simulink model "FOC_Motor_Control"  (R2020b)
settings: Solver=FixedStepDiscrete  StartTime=0.0  StopTime=10.0  FixedStep=Fixed_Step_Size  RelTol=1e-3
values from neighbouring files (symbols this model uses):
  Angle = 1.0    [Hall_Flux_FOC_Data.sldd]    (also in Motor_Control_Data.sldd)
  Cosine_table = 1.0 0.99999529 0.99999058 0.99998587 0.99998116 0.99996704 0.99995291 0.99993885 0.99992472 0.99990118 0.99987763 0.99985409 0.9998306 0.99979764 0.99976468 0.99973178 0.99969882 0.99965644 0.99961412 0.99957174 0.99952942 0.99947762 0.99942589 0.99937415 0.99932235 0.9992612 0.99920005 0.99913889 0.99907768 0.99900717 0.99893659 0.99886602 0.99879545 0.99871546 0.99863547 0.99855554 0.99847555 0.    [Hall_Flux_FOC_Data.sldd]    (also in Motor_Control_Data.sldd)
  Flux = 0.0109    [G474_FOC_LADRC.sldd]    (also in G474_FOC_NONOBSERVER.sldd = 0.0109
  HaLL_AngleShift = -0.25    [Hall_Flux_FOC_Data.sldd]
  HaLL_Sector1 = 5.236    [Hall_Flux_FOC_Data.sldd]
  HaLL_Sector2 = 1.0472    [Hall_Flux_FOC_Data.sldd]
  HaLL_Sector3 = 0.0    [Hall_Flux_FOC_Data.sldd]
  HaLL_Sector4 = 3.1415    [Hall_Flux_FOC_Data.sldd]
  HaLL_Sector5 = 4.1888    [Hall_Flux_FOC_Data.sldd]
  HaLL_Sector6 = 2.0944    [Hall_Flux_FOC_Data.sldd]
  HaLL_Timer_T = 1.0E-5    [Hall_Flux_FOC_Data.sldd]
  ID_Ki = 1.3    [Hall_Flux_FOC_Data.sldd]    (also in Motor_Control_Data.sldd = 48.0
  ID_Kp = 0.4    [Hall_Flux_FOC_Data.sldd]    (also in Motor_Control_Data.sldd = 0.84
  inverter = struct    [PMSM_Parameters.m]
  IQ_Ki = 1.6    [Hall_Flux_FOC_Data.sldd]    (also in Motor_Control_Data.sldd = 48.0
  IQ_Kp = 0.4    [Hall_Flux_FOC_Data.sldd]    (also in Motor_Control_Data.sldd = 1.869
  LADRC_b0 = 10000.0    [G474_FOC_LADRC.sldd]    (also in Hall_Flux_FOC_Data.sldd = 80000.0
  LADRC_Omega_c = 100.0    [G474_FOC_LADRC.sldd]    (also in Hall_Flux_FOC_Data.sldd = 80.0
  Ld = 0.0004    [Hall_Flux_FOC_Data.sldd]    (also in Motor_Control_Data.sldd = 0.00014
  Lq = 0.00045    [Hall_Flux_FOC_Data.sldd]    (also in Motor_Control_Data.sldd = 0.0003115
  OPL_Speed = 800.0    [Hall_Flux_FOC_Data.sldd]
  OPL_Time = 2.0    [Hall_Flux_FOC_Data.sldd]
  OPL_Torque = 3.0    [Hall_Flux_FOC_Data.sldd]
  Over_modulation = 0.0    [Hall_Flux_FOC_Data.sldd]    (also in Motor_Control_Data.sldd)
  pll_omega = 5000.0    [G474_FOC_LADRC.sldd]    (also in G474_FOC_NONOBSERVER.sldd)
  pll_xi = 10.0    [G474_FOC_LADRC.sldd]    (also in G474_FOC_NONOBSERVER.sldd)
  Pole_Pairs = 2.0    [Hall_Flux_FOC_Data.sldd]    (also in Motor_Control_Data.sldd = 4.0
  PWM_Frequency = 10000.0    [Hall_Flux_FOC_Data.sldd]    (also in Motor_Control_Data.sldd = 20000.0
  R = 0.405    [Hall_Flux_FOC_Data.sldd]    (also in Motor_Control_Data.sldd = 0.016
  Sine_table = 0.0 0.0015339879 0.0030679768 0.0046019657 0.0061359555 0.0076698866 0.0092038177 0.010737749 0.012271681 0.013805497 0.015339312 0.016873131 0.018406944 0.019940587 0.021474229 0.023007872 0.024541514 0.026074925 0.027608337 0.029141748 0.03067516 0.032208283 0.033741407 0.035274528 0.036807653 0.038340431 0.039873205 0.04140598 0.042938754 0.04447113 0.046003502 0.047535874 0.049068246 0.0506001    [Hall_Flux_FOC_Data.sldd]    (also in Motor_Control_Data.sldd)
  Speed_Ki = 0.06    [Hall_Flux_FOC_Data.sldd]    (also in Motor_Control_Data.sldd = 10.809
  Speed_Kp = 0.002    [Hall_Flux_FOC_Data.sldd]    (also in Motor_Control_Data.sldd = 0.08
  Speed_PI_OutputMax = 3.0    [Hall_Flux_FOC_Data.sldd]    (also in Motor_Control_Data.sldd = 700.0
  Speed_PI_OutputMin = -5.0    [Hall_Flux_FOC_Data.sldd]    (also in Motor_Control_Data.sldd = -700.0
  SpeedFilter_Fn = 0.3    [Hall_Flux_FOC_Data.sldd]    (also in Motor_Control_Data.sldd = 0.2
  TorqueMode = 0.0    [Hall_Flux_FOC_Data.sldd]    (also in Motor_Control_Data.sldd)
undefined symbols (not defined in the file or in its folder): DiscIntNeverNeededParam, Flux_Gain, Flux_Theta_Enable, magnitude, SVPWM
libraries: simulink x6, dspstat3 x1, pid_lib x1
(part 1 of 3)
settings Model: DataDictionary=Hall_Flux_FOC_Data.sldd  Creator=Administrator  LastModifiedBy=Administrator
settings OptimizationCC: DefaultParameterBehavior=Inlined  UseDivisionForNetSlopeComputation=on  GainParamInheritBuiltInType=on  UseFloatMulNetSlope=on  InlineInvariantSignals=on  PassReuseOutputArgsAs=Individual arguments  ZeroExternalMemoryAtStartup=off  ZeroInternalMemoryAtStartup=off  NoFixptDivByZeroProtection=on  EfficientFloat2IntCast=on  LifeSpan=1  OptimizeBlockOrder=speed  DifferentSizesBufferReuse=on  EfficientTunableParamExpr=on
settings DebuggingCC: ParameterTunabilityLossMsg=error
settings HardwareCC: ProdBitPerPointer=32  ProdBitPerSizeT=32  ProdBitPerPtrDiffT=32  ProdLargestAtomicInteger=Long  ProdLargestAtomicFloat=Double  ProdWordSize=32  ProdLongLongMode=on  ProdHWDeviceType=NXP->Cortex-M4
settings ModelReferenceCC: ModelReferenceNumInstancesAllowed=Single
settings SFSimCC: MATLABDynamicMemAlloc=off
settings RTWCC: Description=Embedded Coder  SystemTargetFile=ert.tlc  GenCodeOnly=on  TemplateMakefile=ert_default_tmf  GenerateReport=on  BuildConfiguration=Faster Runs  LaunchReport=on
settings CodeAppCC: ForceParamTrailComments=on  IgnoreCustomStorageClasses=off  MaxIdLength=64  OperatorAnnotations=on  SimulinkDataObjDesc=on  SFDataObjDesc=on  CustomSymbolStrGlobalVar=rt$N$M  CustomSymbolStrType=$N$M  CustomSymbolStrFcn=$N$M$F  CustomSymbolStrMacro=$N$M  InsertBlockDesc=on
settings ERTTargetCC: TargetLangStandard=C99 (ISO)  GenerateSampleERTMain=on  IncludeMdlTerminateFcn=off  CombineSignalStateStructs=on  SupportAbsoluteTime=off  SupportComplex=off  SupportNonInlinedSFcns=on  InlinedParameterPlacement=NonHierarchical  ERTCustomFileTemplate=example_file_process.tlc

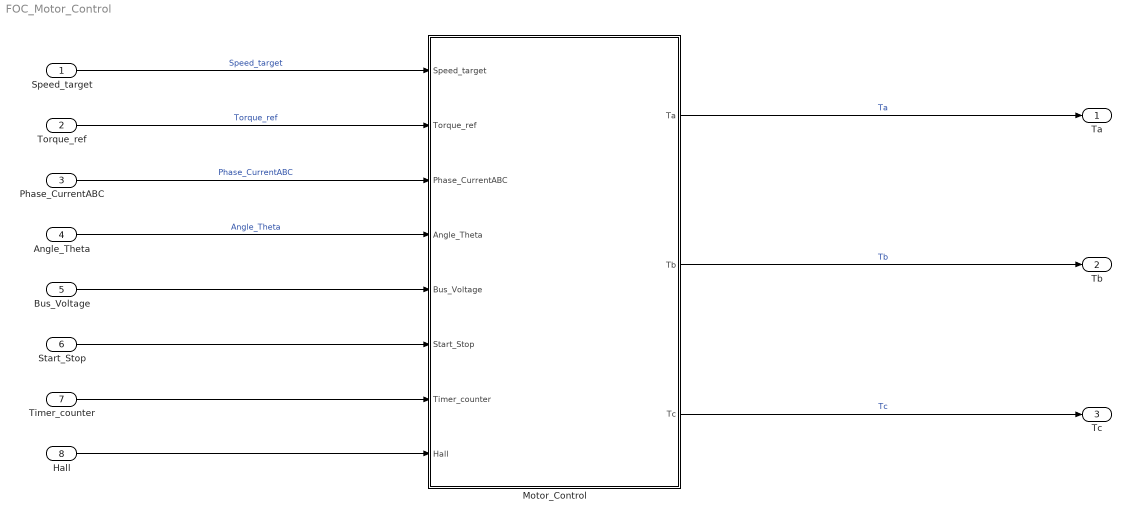
== system FOC_Motor_Control ==
  Speed_target : Inport
  Torque_ref : Inport  Port=2  OutMin=0  OutMax=2*pi  OutDataTypeStr=single
  Phase_CurrentABC : Inport  Port=3  OutDataTypeStr=single  PortDimensions=3
  Angle_Theta : Inport  Port=4  OutMin=0  OutMax=2*pi
  Bus_Voltage : Inport  Port=5
  Start_Stop : Inport  Port=6
  Timer_counter : Inport  Port=7  OutDataTypeStr=single
  Hall : Inport  Port=8
  Motor_Control : Subsystem  TreatAsAtomicUnit=on
  Ta : Outport
  Tb : Outport  Port=2
  Tc : Outport  Port=3
  wires:
  Speed_target/1 -> Motor_Control/1(Speed_target)  "Speed_target"
  Motor_Control/1(Ta) -> Ta/1  "Ta"
  Motor_Control/3(Tc) -> Tc/1  "Tc"
  Motor_Control/2(Tb) -> Tb/1  "Tb"
  Phase_CurrentABC/1 -> Motor_Control/3(Phase_CurrentABC)  "Phase_CurrentABC"
  Angle_Theta/1 -> Motor_Control/4(Angle_Theta)  "Angle_Theta"
  Torque_ref/1 -> Motor_Control/2(Torque_ref)  "Torque_ref"
  Bus_Voltage/1 -> Motor_Control/5(Bus_Voltage)
  Start_Stop/1 -> Motor_Control/6(Start_Stop)
  Hall/1 -> Motor_Control/8(Hall)
  Timer_counter/1 -> Motor_Control/7(Timer_counter)

== system FOC_Motor_Control/Motor_Control ==
  Speed_target : Inport
  Torque_ref : Inport  Port=2  OutMin=0  OutMax=2*pi
  Phase_CurrentABC : Inport  Port=3  PortDimensions=3
  Angle_Theta : Inport  Port=4  OutMin=0  OutMax=2*pi
  Bus_Voltage : Inport  Port=5
  Start_Stop : Inport  Port=6
  Timer_counter : Inport  Port=7
  Hall : Inport  Port=8
  Motor_Control_Function : Subsystem
  Ta : Outport
  Tb : Outport  Port=2
  Tc : Outport  Port=3
  wires:
  Motor_Control_Function/2(Tb) -> Tb/1
  Motor_Control_Function/3(Tc) -> Tc/1
  Motor_Control_Function/1(Ta) -> Ta/1
  Speed_target/1 -> Motor_Control_Function/1(Speed_target)  "Speed_target"
  Phase_CurrentABC/1 -> Motor_Control_Function/2(Phase_CurrentABC)  "Phase_CurrentABC"
  Angle_Theta/1 -> Motor_Control_Function/3(Angle_Theta)  "Angle_Theta"
  Start_Stop/1 -> Motor_Control_Function/5(Start_Stop)
  Bus_Voltage/1 -> Motor_Control_Function/4(Bus_voltage)
  Torque_ref/1 -> Motor_Control_Function/6(Torque_ref)
  Timer_counter/1 -> Motor_Control_Function/7(Timer_counter)
  Hall/1 -> Motor_Control_Function/8(Hall)

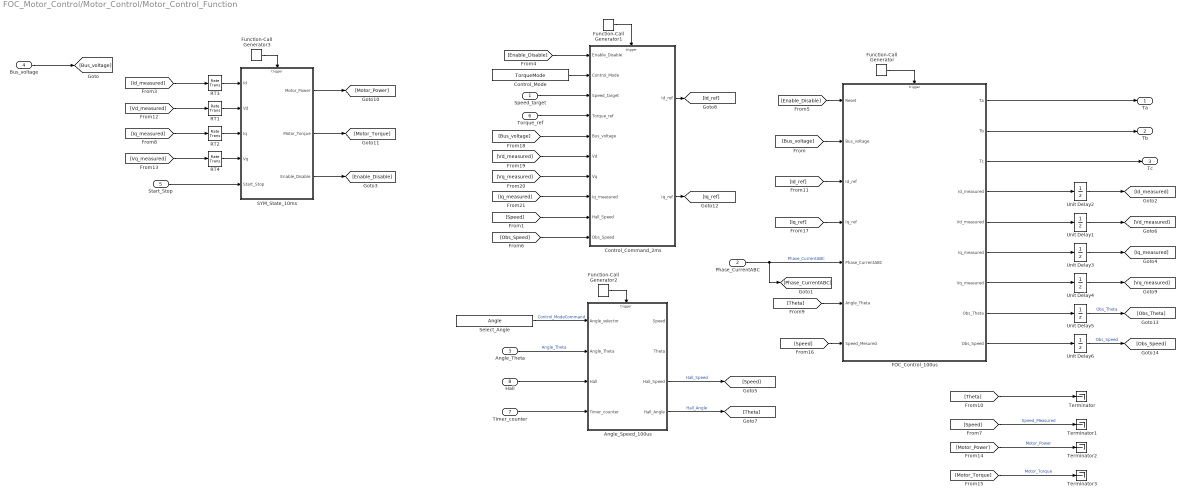
== system FOC_Motor_Control/Motor_Control/Motor_Control_Function ==
  Speed_target : Inport
  Phase_CurrentABC : Inport  Port=2  PortDimensions=3
  Angle_Theta : Inport  Port=3  OutMin=0  OutMax=2*pi
  Bus_voltage : Inport  Port=4
  Start_Stop : Inport  Port=5
  Torque_ref : Inport  Port=6  OutMin=0  OutMax=2*pi
  Timer_counter : Inport  Port=7
  Hall : Inport  Port=8
  Angle_Speed_100us : Subsystem
      settings: RTWSystemCode=Nonreusable function  RTWFcnNameOpts=Use subsystem name  RTWFileNameOpts=Use subsystem name
  Control_Command_2ms : Subsystem  TreatAsAtomicUnit=on
      settings: RTWSystemCode=Nonreusable function  RTWFcnNameOpts=Use subsystem name  RTWFileNameOpts=Use subsystem name  FunctionInterfaceSpec=Allow arguments (Optimized)
  Control_Mode : Constant  Value=TorqueMode
  FOC_Control_100us : Subsystem  TreatAsAtomicUnit=on
      settings: RTWSystemCode=Nonreusable function  RTWFcnNameOpts=Use subsystem name  RTWFileNameOpts=Use subsystem name  FunctionInterfaceSpec=Allow arguments (Optimized)
  Function-Call Generator : simulink/Ports & Subsystems/Function-Call Generator  sample_time=1/PWM_Frequency  numberOfIterations=1  DisallowWideOutput=off
  Function-Call Generator1 : simulink/Ports & Subsystems/Function-Call Generator  sample_time=Task_2ms  numberOfIterations=1  DisallowWideOutput=off
  Function-Call Generator2 : simulink/Ports & Subsystems/Function-Call Generator  sample_time=1/PWM_Frequency  numberOfIterations=1  DisallowWideOutput=off
  Function-Call Generator3 : simulink/Ports & Subsystems/Function-Call Generator  sample_time=Task_10ms  numberOfIterations=1  DisallowWideOutput=off
  RT{1..4} (4 alike) : RateTransition  Integrity=off
  SYM_State_10ms : Subsystem
      settings: RTWSystemCode=Nonreusable function  RTWFcnNameOpts=Use subsystem name  RTWFileNameOpts=Use subsystem name
  Select_Angle : Constant  Value=Angle
  Terminator{,1..3} (4 alike) : Terminator
  Unit Delay{1..6} (6 alike) : UnitDelay  SampleTime=-1  HasFrameUpgradeWarning=on
  Ta : Outport
  Tb : Outport  Port=2
  Tc : Outport  Port=3
  wires:
  Function-Call Generator1/1 -> Control_Command_2ms/Trigger
  Control_Mode/1 -> Control_Command_2ms/2(Control_Mode)
  Angle_Theta/1 -> Angle_Speed_100us/2(Angle_Theta)  "Angle_Theta"
  Function-Call Generator/1 -> FOC_Control_100us/Trigger
  Phase_CurrentABC/1 -> FOC_Control_100us/5(Phase_CurrentABC), [Phase_CurrentABC]  "Phase_CurrentABC"
  FOC_Control_100us/3(Tc) -> Tc/1
  Select_Angle/1 -> Angle_Speed_100us/1(Angle_selector)  "Control_ModeCommand"
  Speed_target/1 -> Control_Command_2ms/3(Speed_target)
  FOC_Control_100us/2(Tb) -> Tb/1
  FOC_Control_100us/1(Ta) -> Ta/1
  Function-Call Generator2/1 -> Angle_Speed_100us/Trigger
  Function-Call Generator3/1 -> SYM_State_10ms/Trigger
  SYM_State_10ms/3(Enable_Disable) -> [Enable_Disable]
  [Enable_Disable] -> Control_Command_2ms/1(Enable_Disable)
  [Enable_Disable] -> FOC_Control_100us/1(Reset)
  [Speed] -> Terminator1/1  "Speed_Measured"
  [Theta] -> FOC_Control_100us/6(Angle_Theta)
  [Theta] -> Terminator/1
  Control_Command_2ms/1(Id_ref) -> [Id_ref]
  [Id_ref] -> FOC_Control_100us/3(Id_ref)
  Start_Stop/1 -> SYM_State_10ms/5(Start_Stop)
  Bus_voltage/1 -> [Bus_voltage]
  FOC_Control_100us/6(Iq_measured) -> Unit Delay3/1
  FOC_Control_100us/7(Vq_measured) -> Unit Delay4/1
  FOC_Control_100us/4(Id_measured) -> Unit Delay2/1
  FOC_Control_100us/5(Vd_measured) -> Unit Delay1/1
  Unit Delay2/1 -> [Id_measured]
  Unit Delay1/1 -> [Vd_measured]
  Unit Delay3/1 -> [Iq_measured]
  Unit Delay4/1 -> [Vq_measured]
  [Iq_measured] -> RT2/1
  [Id_measured] -> RT3/1
  [Vd_measured] -> RT1/1
  [Vq_measured] -> RT4/1
  SYM_State_10ms/1(Motor_Power) -> [Motor_Power]
  [Motor_Power] -> Terminator2/1  "Motor_Power"
  RT3/1 -> SYM_State_10ms/1(Id)
  RT1/1 -> SYM_State_10ms/2(Vd)
  RT2/1 -> SYM_State_10ms/3(Iq)
  RT4/1 -> SYM_State_10ms/4(Vq)
  [Bus_voltage] -> FOC_Control_100us/2(Bus_voltage)
  SYM_State_10ms/2(Motor_Torque) -> [Motor_Torque]
  [Motor_Torque] -> Terminator3/1  "Motor_Torque"
  Torque_ref/1 -> Control_Command_2ms/4(Torque_ref)
  [Speed] -> FOC_Control_100us/7(Speed_Mesured)
  [Obs_Speed] -> Control_Command_2ms/10(Obs_Speed)
  Control_Command_2ms/2(Iq_ref) -> [Iq_ref]
  [Iq_ref] -> FOC_Control_100us/4(Iq_ref)
  [Bus_voltage] -> Control_Command_2ms/5(Bus_voltage)
  [Vd_measured] -> Control_Command_2ms/6(Vd)
  [Vq_measured] -> Control_Command_2ms/7(Vq)
  [Iq_measured] -> Control_Command_2ms/8(Iq_measured)
  Hall/1 -> Angle_Speed_100us/3(Hall)
  Timer_counter/1 -> Angle_Speed_100us/4(Timer_counter)
  FOC_Control_100us/8(Obs_Theta) -> Unit Delay5/1
  FOC_Control_100us/9(Obs_Speed) -> Unit Delay6/1
  Unit Delay5/1 -> [Obs_Theta]  "Obs_Theta"
  Unit Delay6/1 -> [Obs_Speed]  "Obs_Speed"
  [Speed] -> Control_Command_2ms/9(Hall_Speed)
  Angle_Speed_100us/3(Hall_Speed) -> [Speed]  "Hall_Speed"
  Angle_Speed_100us/4(Hall_Angle) -> [Theta]  "Hall_Angle"

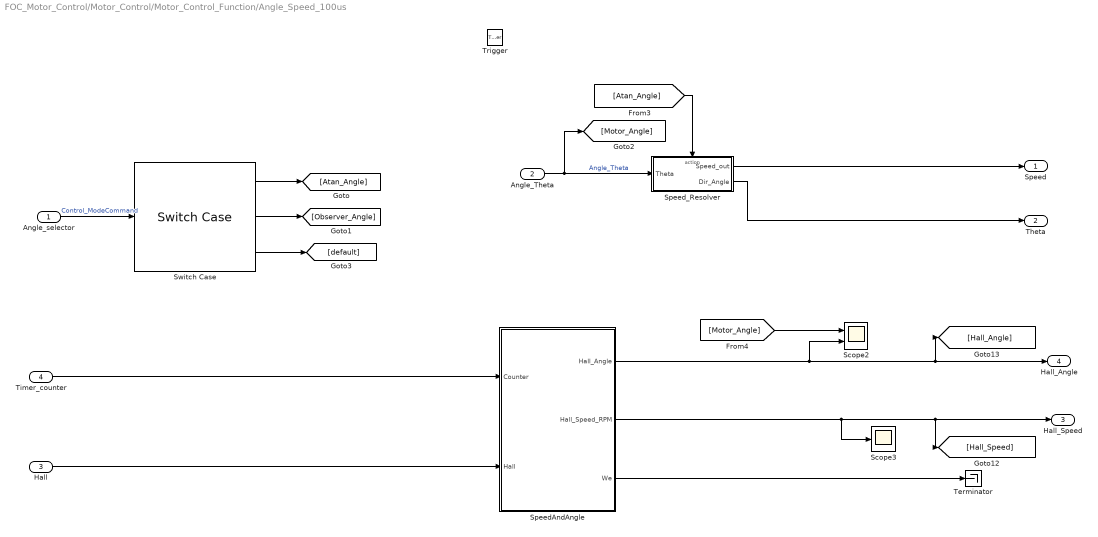
== system FOC_Motor_Control/Motor_Control/Motor_Control_Function/Angle_Speed_100us ==
  Angle_selector : Inport
  Angle_Theta : Inport  Port=2  OutMin=0  OutMax=2*pi
  Hall : Inport  Port=3
  Timer_counter : Inport  Port=4
  Trigger : TriggerPort  TriggerType=function-call  VariantControl=Variant  SampleTimeType=periodic  SampleTime=-1  PortDimensions=1
  Scope2 : Scope  NumInputPorts=2
  Scope3 : Scope
  SpeedAndAngle : Subsystem
      settings: RTWSystemCode=Nonreusable function  RTWFcnNameOpts=Use subsystem name  RTWFileNameOpts=Use subsystem name
  Speed_Resolver : Subsystem  TreatAsAtomicUnit=on
      settings: RTWSystemCode=Nonreusable function  RTWFcnNameOpts=Use subsystem name
  Switch Case : SwitchCase  CaseConditions={1,2}
  Terminator : Terminator
  Speed : Outport
  Theta : Outport  Port=2
  Hall_Speed : Outport  Port=3
  Hall_Angle : Outport  Port=4
  wires:
  Speed_Resolver/1(Speed_out) -> Speed/1
  Speed_Resolver/2(Dir_Angle) -> Theta/1
  Angle_selector/1 -> Switch Case/1  "Control_ModeCommand"
  Switch Case/3 -> [default]
  Switch Case/1 -> [Atan_Angle]
  Switch Case/2 -> [Observer_Angle]
  Angle_Theta/1 -> [Motor_Angle], Speed_Resolver/1(Theta)  "Angle_Theta"
  [Atan_Angle] -> Speed_Resolver/Action
  SpeedAndAngle/1(Hall_Angle) -> Scope2/2, [Hall_Angle], Hall_Angle/1
  SpeedAndAngle/3(We) -> Terminator/1
  Hall/1 -> SpeedAndAngle/2(Hall)
  Timer_counter/1 -> SpeedAndAngle/1(Counter)
  [Motor_Angle] -> Scope2/1
  SpeedAndAngle/2(Hall_Speed_RPM) -> Hall_Speed/1, [Hall_Speed], Scope3/1

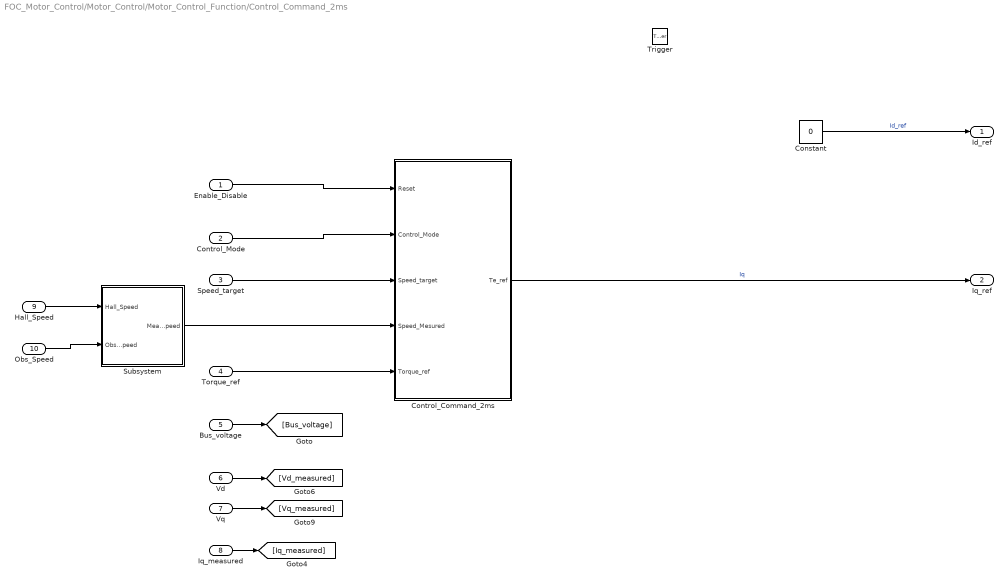
== system FOC_Motor_Control/Motor_Control/Motor_Control_Function/Control_Command_2ms ==
  Enable_Disable : Inport
  Control_Mode : Inport  Port=2
  Speed_target : Inport  Port=3
  Torque_ref : Inport  Port=4  OutMin=0  OutMax=2*pi
  Bus_voltage : Inport  Port=5
  Vd : Inport  Port=6
  Vq : Inport  Port=7
  Iq_measured : Inport  Port=8
  Hall_Speed : Inport  Port=9  OutMin=0  OutMax=2*pi
  Obs_Speed : Inport  Port=10  OutMin=0  OutMax=2*pi
  Trigger : TriggerPort  TriggerType=function-call  VariantControl=Variant  SampleTimeType=periodic  SampleTime=-1  PortDimensions=1
  Constant : Constant  Value=0  OutDataTypeStr=single
  Control_Command_2ms : Subsystem  TreatAsAtomicUnit=on
      settings: RTWSystemCode=Nonreusable function  RTWFcnNameOpts=Use subsystem name  RTWFileNameOpts=Use subsystem name  FunctionInterfaceSpec=Allow arguments (Optimized)
  Subsystem : Subsystem
  Id_ref : Outport
  Iq_ref : Outport  Port=2
  wires:
  Control_Mode/1 -> Control_Command_2ms/2(Control_Mode)
  Speed_target/1 -> Control_Command_2ms/3(Speed_target)
  Enable_Disable/1 -> Control_Command_2ms/1(Reset)
  Torque_ref/1 -> Control_Command_2ms/5(Torque_ref)
  Control_Command_2ms/1(Te_ref) -> Iq_ref/1  "Iq"
  Constant/1 -> Id_ref/1  "Id_ref"
  Bus_voltage/1 -> [Bus_voltage]
  Vd/1 -> [Vd_measured]
  Vq/1 -> [Vq_measured]
  Iq_measured/1 -> [Iq_measured]
  Subsystem/1(Measured_Speed) -> Control_Command_2ms/4(Speed_Mesured)
  Hall_Speed/1 -> Subsystem/1(Hall_Speed)
  Obs_Speed/1 -> Subsystem/2(Obs_Speed)

== system FOC_Motor_Control/Motor_Control/Motor_Control_Function/FOC_Control_100us ==
  Reset : Inport
  Bus_voltage : Inport  Port=2
  Id_ref : Inport  Port=3
  Iq_ref : Inport  Port=4
  Phase_CurrentABC : Inport  Port=5  PortDimensions=3
  Angle_Theta : Inport  Port=6  OutMin=0  OutMax=2*pi
  Speed_Mesured : Inport  Port=7  OutMin=0  OutMax=2*pi
  Trigger : TriggerPort  TriggerType=function-call  VariantControl=Variant  SampleTimeType=periodic  SampleTime=-1  PortDimensions=1
  FOC : Subsystem  TreatAsAtomicUnit=on
      settings: RTWSystemCode=Nonreusable function  RTWFcnNameOpts=Use subsystem name
  Ta : Outport
  Tb : Outport  Port=2
  Tc : Outport  Port=3
  Id_measured : Outport  Port=4
  Vd_measured : Outport  Port=5
  Iq_measured : Outport  Port=6
  Vq_measured : Outport  Port=7
  Obs_Theta : Outport  Port=8
  Obs_Speed : Outport  Port=9
  wires:
  FOC/1(Ta) -> Ta/1  "Ta"
  FOC/2(Tb) -> Tb/1  "Tb"
  FOC/3(Tc) -> Tc/1  "Tc"
  Angle_Theta/1 -> FOC/5(Angle_Theta)  "Angle_Theta"
  Phase_CurrentABC/1 -> FOC/6(Phase_CurrentABC)  "Phase_CurrentABC"
  Reset/1 -> FOC/1(Reset)
  FOC/6(Iq_measured) -> Iq_measured/1
  FOC/7(Vq_measured) -> Vq_measured/1
  FOC/4(Id_measured) -> Id_measured/1
  FOC/5(Vd_measured) -> Vd_measured/1
  Bus_voltage/1 -> FOC/2(Bus_voltage)
  Speed_Mesured/1 -> FOC/7(Speed_Mesured)  "Speed_Measured"
  Id_ref/1 -> FOC/3(Id_target)  "Id_ref"
  Iq_ref/1 -> FOC/4(Iq_target)  "Iq_ref"
  FOC/8(Obs_Theta) -> Obs_Theta/1
  FOC/9(Obs_Speed) -> Obs_Speed/1

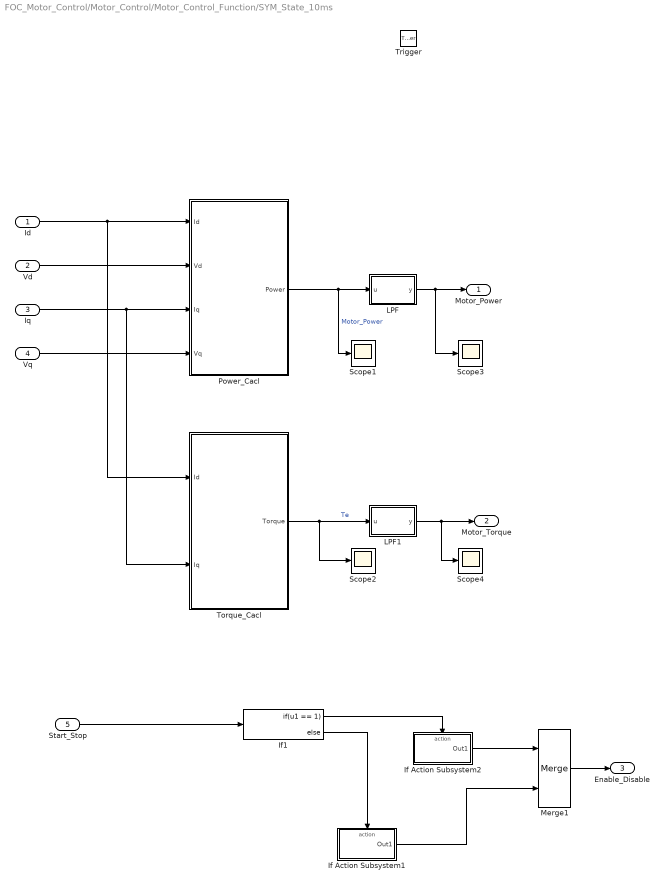
== system FOC_Motor_Control/Motor_Control/Motor_Control_Function/SYM_State_10ms ==
  Id : Inport
  Vd : Inport  Port=2
  Iq : Inport  Port=3
  Vq : Inport  Port=4
  Start_Stop : Inport  Port=5  OutDataTypeStr=uint8
  Trigger : TriggerPort  TriggerType=function-call  VariantControl=Variant  SampleTimeType=periodic  SampleTime=-1  PortDimensions=1
  If Action Subsystem1 : Subsystem  TreatAsAtomicUnit=on
  If Action Subsystem2 : Subsystem  TreatAsAtomicUnit=on
  If1 : If  IfExpression=u1 == 1
  LPF : Subsystem
  LPF1 : Subsystem
  Merge1 : Merge
  Power_Cacl : Subsystem
  Scope{1..4} (4 alike) : Scope
  Torque_Cacl : Subsystem
  Motor_Power : Outport
  Motor_Torque : Outport  Port=2
  Enable_Disable : Outport  Port=3
  wires:
  Iq/1 -> Torque_Cacl/2(Iq), Power_Cacl/3(Iq)
  Vq/1 -> Power_Cacl/4(Vq)
  Power_Cacl/1(Power) -> LPF/1(u), Scope1/1  "Motor_Power"
  Vd/1 -> Power_Cacl/2(Vd)
  Id/1 -> Torque_Cacl/1(Id), Power_Cacl/1(Id)
  LPF/1(y) -> Scope3/1, Motor_Power/1
  Torque_Cacl/1(Torque) -> LPF1/1(u), Scope2/1  "Te"
  LPF1/1(y) -> Motor_Torque/1, Scope4/1
  Start_Stop/1 -> If1/1
  If1/2 -> If Action Subsystem1/Action
  If1/1 -> If Action Subsystem2/Action
  If Action Subsystem2/1(Out1) -> Merge1/1
  If Action Subsystem1/1(Out1) -> Merge1/2
  Merge1/1 -> Enable_Disable/1

== system FOC_Motor_Control/Motor_Control/Motor_Control_Function/Angle_Speed_100us/SpeedAndAngle ==
  Counter : Inport
  Hall : Inport  Port=2  OutDataTypeStr=uint8
  ACC_OMG : Subsystem  TreatAsAtomicUnit=on
      settings: RTWSystemCode=Nonreusable function  RTWFcnNameOpts=Use subsystem name
  ADC_IRQ : Subsystem  TreatAsAtomicUnit=on
      settings: RTWSystemCode=Nonreusable function  RTWFcnNameOpts=Use subsystem name
  Scope : Scope
  Hall_Angle : Outport
  Hall_Speed_RPM : Outport  Port=2
  We : Outport  Port=3
  wires:
  ACC_OMG/4(Counter) -> ADC_IRQ/4(Counter_Hall_IRQ)
  ACC_OMG/2(Acc) -> ADC_IRQ/2(Acc)
  ACC_OMG/3(OMG) -> We/1, ADC_IRQ/3(OMG), [Hall_We]
  ACC_OMG/1(Hall_SpeedRPM) -> Hall_Speed_RPM/1
  ACC_OMG/5(Six_theta) -> ADC_IRQ/5(Six_theta)
  Counter/1 -> ADC_IRQ/1(Counter_ADC_IRQ), ACC_OMG/1(Timer_Counter)
  ADC_IRQ/1(Hall_Angle) -> Hall_Angle/1, Scope/1
  Hall/1 -> ACC_OMG/2(Hall), ACC_OMG/Trigger

== system FOC_Motor_Control/Motor_Control/Motor_Control_Function/Angle_Speed_100us/Speed_Resolver ==
  Theta : Inport
  Action Port : ActionPort  ActionPortLabel=case [ 1 ]:
  DT2 : DataTypeConversion  OutDataTypeStr=single
  Speed_cacl : Subsystem  TreatAsAtomicUnit=on
      settings: RTWSystemCode=Nonreusable function  RTWFcnNameOpts=Use subsystem name
  Speed_out : Outport
  Dir_Angle : Outport  Port=2
  wires:
  Theta/1 -> DT2/1, Speed_cacl/1(position)
  Speed_cacl/1(Speed_RPM) -> Speed_out/1  "Speed_Measured"
  DT2/1 -> Dir_Angle/1  "Direct_Angle"

== system FOC_Motor_Control/Motor_Control/Motor_Control_Function/Control_Command_2ms/Control_Command_2ms ==
  Reset : Inport
  Control_Mode : Inport  Port=2
  Speed_target : Inport  Port=3
  Speed_Mesured : Inport  Port=4  OutMin=0  OutMax=2*pi
  Torque_ref : Inport  Port=5  OutMin=0  OutMax=2*pi
  Merge : Merge
  Speed_PI : Subsystem  TreatAsAtomicUnit=on  SystemSampleTime=inverter.Ts
      settings: RTWSystemCode=Nonreusable function
  Switch Case : SwitchCase  CaseConditions={0,1}
  Switch Case Action Subsystem : Subsystem  TreatAsAtomicUnit=on
      settings: RTWSystemCode=Nonreusable function
  Te_ref : Outport
  wires:
  Switch Case Action Subsystem/1(Iq_out) -> Merge/2
  Torque_ref/1 -> Switch Case Action Subsystem/1(Iq_in)
  Switch Case/3 -> [default]
  [Torque_Mode] -> Switch Case Action Subsystem/Action
  Switch Case/2 -> [Torque_Mode]
  Switch Case/1 -> [Speed_Mode]
  Control_Mode/1 -> Switch Case/1
  [Speed_Mode] -> Speed_PI/Action
  Speed_PI/1(Iq_ref) -> Merge/1  "Iq_ref"
  Merge/1 -> Te_ref/1
  Speed_target/1 -> Speed_PI/1(Speed_Command)
  Reset/1 -> Speed_PI/3(Reset)
  Speed_Mesured/1 -> Speed_PI/2(Speed_Measured)

== system FOC_Motor_Control/Motor_Control/Motor_Control_Function/Control_Command_2ms/Subsystem ==
  Hall_Speed : Inport
  Obs_Speed : Inport  Port=2
  Flux_Enable : Constant  Value=Flux_Theta_Enable  OutDataTypeStr=uint8
  Hall_Spd : Subsystem  TreatAsAtomicUnit=on
  If1 : If  IfExpression=u1==1  ElseIfExpressions=u1==0  ShowElse=off
  Merge : Merge
  Obs_Spd : Subsystem  TreatAsAtomicUnit=on
  Measured_Speed : Outport
  wires:
  If1/1 -> Obs_Spd/Action
  Hall_Spd/1(Out1) -> Merge/2
  Merge/1 -> Measured_Speed/1
  Hall_Speed/1 -> Hall_Spd/1(Hall_Speed)
  Obs_Spd/1(Out1) -> Merge/1
  If1/2 -> Hall_Spd/Action
  Obs_Speed/1 -> Obs_Spd/1(Obs_Speed)
  Flux_Enable/1 -> If1/1

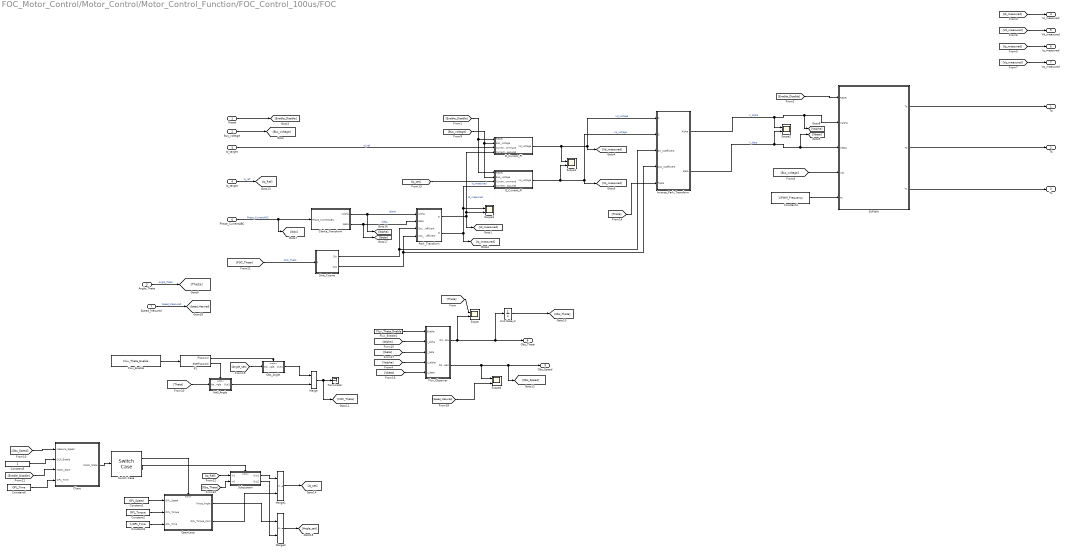
== system FOC_Motor_Control/Motor_Control/Motor_Control_Function/FOC_Control_100us/FOC ==
  Reset : Inport
  Bus_voltage : Inport  Port=2
  Id_target : Inport  Port=3
  Iq_target : Inport  Port=4
  Angle_Theta : Inport  Port=5  OutMin=0  OutMax=2*pi
  Phase_CurrentABC : Inport  Port=6  PortDimensions=3
  Speed_Mesured : Inport  Port=7  OutMin=0  OutMax=2*pi
  Chart : Stateflow chart  TreatAsAtomicUnit=on
  Clarke_Transform : Subsystem  TreatAsAtomicUnit=on
      settings: RTWSystemCode=Nonreusable function  RTWFcnNameOpts=Use subsystem name
  Constant1 : Constant  Value=OPL_Speed  OutDataTypeStr=single
  Constant2 : Constant  Value=OPL_Torque
  Constant3 : Constant  Value=1/OPL_Time
  Constant4 : Constant  Value=1/PWM_Frequency  OutDataTypeStr=single
  Constant5 : Constant  OutDataTypeStr=uint8
  Constant6 : Constant  Value=OPL_Time
  D_Current_PI : Subsystem  TreatAsAtomicUnit=on
      settings: RTWSystemCode=Nonreusable function  RTWFcnNameOpts=Use subsystem name
  Flux_Enable : Constant  Value=Flux_Theta_Enable  OutDataTypeStr=uint8
  Flux_Enable1 : Constant  Value=Flux_Theta_Enable  OutDataTypeStr=uint8
  Flux_Observer : Subsystem
  Hall_Angle : Subsystem  TreatAsAtomicUnit=on
  If1 : If  IfExpression=u1==1  ElseIfExpressions=u1==0  ShowElse=off
  Inverse_Park_Transform : Subsystem  TreatAsAtomicUnit=on
      settings: RTWSystemCode=Nonreusable function  RTWFcnNameOpts=Use subsystem name
      mask Display:
      | port_label('input',1,'D')
      | port_label('input',2,'Q')
      | port_label('input',3,'Sin')
      | port_label('input',4,'Cos')
      | port_label('output',1,'\alpha','texmode', 'on')
      | port_label('output',2,'\beta','texmode', 'on')
  Merge : Merge
  Merge1 : Merge
  Merge2 : Merge
  Obs_Angle : Subsystem  TreatAsAtomicUnit=on
  OpenLoop : Subsystem
  Park_Transform : Subsystem  TreatAsAtomicUnit=on
      settings: RTWSystemCode=Nonreusable function  RTWFcnNameOpts=Use subsystem name
      mask Display:
      | port_label('input',1,'\alpha','texmode', 'on')
      | port_label('input',2,'\beta','texmode', 'on')
      | port_label('input',3,'Sin')
      | port_label('input',4,'Cos')
      | port_label('output',1,'D')
      | port_label('output',2,'Q')
  Q_Current_PI : Subsystem  TreatAsAtomicUnit=on
      settings: RTWSystemCode=Nonreusable function  RTWFcnNameOpts=Use subsystem name
  SVPWM : Subsystem  AncestorBlock=SVPWM/SVPWM  TreatAsAtomicUnit=on  RTWFcnName=SVPWM  RTWFileName=SVPWM
      settings: RTWSystemCode=Nonreusable function  RTWFcnNameOpts=Use subsystem name
      mask Display:
      | plot([0.000 0.020 0.041 0.061 0.082 0.102 0.122 0.143 0.163 0.184 0.204 0.224 0.245 0.265 0.286 0.306 0.327 0.347 0.367 0.388 0.408 0.429 0.449 0.469 0.490 0.510 0.531 0.551 0.571 0.592 0.612 0.633 0.653 0.673 0.694 0.714 0.735 0.755 0.776 0.796 0.816 0.837 0.857 0.878 0.898 0.918 0.939 0.959 0.980 1.000 ], ...
      |      [0.500 0.586 0.671 0.753 0.831 0.858 0.875 0.885 0.890 0.887 0.879 0.864 0.844 0.855 0.872 0.884 0.889 0.888 0.881 0.867 0.847 0.793 0.713 0.629 0.543 0.457 0.371 0.287 0.207 0.153 0.133 0.119 0.112 0.111 0.116 0.128 0.145 0.156 0.136 0.121 0.113 0.110 0.115 0.125 0.142 0.169 0.247 0.329 0.414 0.500 ])
  Scope{,1..4} (5 alike) : Scope  NumInputPorts=2
  Sine_Cosine : Subsystem  TreatAsAtomicUnit=on
      settings: RTWSystemCode=Nonreusable function  RTWFcnNameOpts=Use subsystem name
  Subsystem : Subsystem
  Switch Case : SwitchCase  CaseConditions={1,2}  ShowDefaultCase=off
  Terminator : Terminator
  Unit Delay2 : UnitDelay  SampleTime=-1  HasFrameUpgradeWarning=on
  Ta : Outport
  Tb : Outport  Port=2
  Tc : Outport  Port=3
  Id_measured : Outport  Port=4
  Vd_measured : Outport  Port=5
  Iq_measured : Outport  Port=6
  Vq_measured : Outport  Port=7
  Obs_Theta : Outport  Port=8
  Obs_Speed : Outport  Port=9
  wires:
  Park_Transform/1(D) -> Scope3/2, D_Current_PI/4(Current_Measured), [Id_measured]  "Id_measured"
  Constant4/1 -> SVPWM/5(Ts)
  Park_Transform/2(Q) -> Q_Current_PI/4(Current_Measured), Scope3/1, [Iq_measured]  "Iq_measured"
  Sine_Cosine/2(Cos) -> Park_Transform/4(Cos_Coefficient), Inverse_Park_Transform/4(Cos_Coefficient)
  Sine_Cosine/1(Sin) -> Park_Transform/3(Sin_Coefficient), Inverse_Park_Transform/3(Sin_Coefficient)
  [Bus_voltage] -> SVPWM/4(Vdc)
  D_Current_PI/1(Vd_voltage) -> Scope1/1, [Vd_measured], Inverse_Park_Transform/1(D)  "Vd_voltage"
  Q_Current_PI/1(Vq_voltage) -> Scope1/2, [Vq_measured], Inverse_Park_Transform/2(Q)  "Vq_voltage"
  Clarke_Transform/2(IBeta) -> [Ibeta], Park_Transform/2(Beta)  "Ibeta"
  Clarke_Transform/1(IAlpha) -> Park_Transform/1(Alpha), [Ialpha]  "Ialpha"
  Phase_CurrentABC/1 -> [Iabc], Clarke_Transform/1(Phase_CurrentABC)  "Phase_CurrentABC"
  Angle_Theta/1 -> [Theta]  "Angle_Theta"
  Id_target/1 -> D_Current_PI/3(Current_Command)  "Id_ref"
  Reset/1 -> [Enable_Disable]
  [Enable_Disable] -> D_Current_PI/1(Reset), Q_Current_PI/1(Reset)
  [Enable_Disable] -> SVPWM/1(Reset)
  [Iq_measured] -> Iq_measured/1
  [Id_measured] -> Id_measured/1
  [Vd_measured] -> Vd_measured/1
  [Vq_measured] -> Vq_measured/1
  Bus_voltage/1 -> [Bus_voltage]
  [Bus_voltage] -> D_Current_PI/2(Bus_voltage), Q_Current_PI/2(Bus_voltage)
  SVPWM/1(Ta) -> Ta/1
  SVPWM/2(Tb) -> Tb/1
  SVPWM/3(Tc) -> Tc/1
  Inverse_Park_Transform/1(Alpha) -> [Valpha], SVPWM/2(Valpha), Scope2/1  "V_alpha"
  Inverse_Park_Transform/2(Beta) -> [Vbeta], SVPWM/3(Vbeta), Scope2/2  "V_beta"
  Speed_Mesured/1 -> [Speed_Mesured]  "Speed_Measured"
  [Theta] -> Inverse_Park_Transform/5(Theta)
  [Valpha] -> Flux_Observer/4(u_alpha)
  [Vbeta] -> Flux_Observer/5(u_beta)
  [Ialpha] -> Flux_Observer/2(i_alpha)
  [Ibeta] -> Flux_Observer/3(i_beta)
  Flux_Observer/1(Obs_Theta) -> Scope/2, Unit Delay2/1, Obs_Theta/1
  [Theta] -> Scope/1
  Flux_Enable/1 -> If1/1
  If1/1 -> Obs_Angle/Action
  If1/2 -> Hall_Angle/Action
  [Theta] -> Hall_Angle/1(Hall_Angle)
  [Angle_set] -> Obs_Angle/1(Obs_Angle)
  Obs_Angle/1(Out1) -> Merge/1
  Hall_Angle/1(Out1) -> Merge/2
  Merge/1 -> [FOC_Theta], Terminator/1
  Unit Delay2/1 -> [Obs_Theta]
  Flux_Observer/2(Obs_Speed) -> Scope4/1, [Obs_Speed], Obs_Speed/1
  Flux_Enable1/1 -> Flux_Observer/1(Enable)
  [Speed_Mesured] -> Scope4/2
  Constant1/1 -> OpenLoop/1(OPL_Speed)
  Constant2/1 -> OpenLoop/2(OPL_Torque)
  Constant3/1 -> OpenLoop/3(OPL_Time)
  [Obs_Speed] -> Chart/1(Measure_Speed)
  Constant5/1 -> Chart/2(OLP_Enable)
  [Enable_Disable] -> Chart/3(Motor_Start)
  Chart/1(Motor_State) -> Switch Case/1
  Switch Case/1 -> OpenLoop/Action
  Switch Case/2 -> Subsystem/Action
  Iq_target/1 -> [Iq_Ref]  "Iq_ref"
  [Iq_Ref] -> Subsystem/1(In1)
  Subsystem/1(Out1) -> Merge1/1
  OpenLoop/2(OPL_Torque_Com) -> Merge1/2
  Merge1/1 -> [Iq_set]
  [Iq_set] -> Q_Current_PI/3(Current_Command)
  OpenLoop/1(Force_Angle) -> Merge2/1
  [Obs_Theta] -> Subsystem/2(In2)
  Subsystem/2(Out2) -> Merge2/2
  Merge2/1 -> [Angle_set]
  Constant6/1 -> Chart/4(OPL_Time)
  [FOC_Theta] -> Sine_Cosine/1(P)  "FOC_Theta"

== system FOC_Motor_Control/Motor_Control/Motor_Control_Function/SYM_State_10ms/If Action Subsystem1 ==
  Action Port : ActionPort  ActionPortLabel=else
  Disable : Constant  OutDataTypeStr=uint8
  Out1 : Outport
  wires:
  Disable/1 -> Out1/1

== system FOC_Motor_Control/Motor_Control/Motor_Control_Function/SYM_State_10ms/If Action Subsystem2 ==
  Action Port : ActionPort  ActionPortLabel=if(u1 == 1)
  enable : Constant  Value=0  OutDataTypeStr=uint8
  Out1 : Outport
  wires:
  enable/1 -> Out1/1

== system FOC_Motor_Control/Motor_Control/Motor_Control_Function/SYM_State_10ms/LPF ==
  u : Inport
  Add : Sum  Inputs=+-
  Add1 : Sum
  Constant1 : Constant  Value=0.005  OutDataTypeStr=single
  Divide1 : Product  Inputs=**
  Unit Delay : UnitDelay  SampleTime=-1  HasFrameUpgradeWarning=on
  y : Outport
  wires:
  Constant1/1 -> Divide1/1
  u/1 -> Add/1
  Add/1 -> Divide1/2
  Divide1/1 -> Add1/1
  Unit Delay/1 -> Add/2, Add1/2
  Add1/1 -> Unit Delay/1, y/1

== system FOC_Motor_Control/Motor_Control/Motor_Control_Function/SYM_State_10ms/LPF1 ==
  u : Inport
  Add : Sum  Inputs=+-
  Add1 : Sum
  Constant1 : Constant  Value=0.005  OutDataTypeStr=single
  Divide1 : Product  Inputs=**
  Unit Delay : UnitDelay  SampleTime=-1  HasFrameUpgradeWarning=on
  y : Outport
  wires:
  Constant1/1 -> Divide1/1
  u/1 -> Add/1
  Add/1 -> Divide1/2
  Divide1/1 -> Add1/1
  Unit Delay/1 -> Add/2, Add1/2
  Add1/1 -> Unit Delay/1, y/1

== system FOC_Motor_Control/Motor_Control/Motor_Control_Function/SYM_State_10ms/Power_Cacl ==
  Id : Inport
  Vd : Inport  Port=2
  Iq : Inport  Port=3
  Vq : Inport  Port=4
  Add : Sum
  Product : Product
  Product1 : Product
  Power : Outport
  wires:
  Id/1 -> Product/1
  Vd/1 -> Product/2
  Iq/1 -> Product1/1
  Vq/1 -> Product1/2
  Product/1 -> Add/1
  Product1/1 -> Add/2
  Add/1 -> Power/1

== system FOC_Motor_Control/Motor_Control/Motor_Control_Function/SYM_State_10ms/Torque_Cacl ==
  Id : Inport
  Iq : Inport  Port=2
  Constant : Constant  Value=3/2  OutDataTypeStr=single
  Constant1 : Constant  Value=Pole_Pairs  OutDataTypeStr=single
  Constant2 : Constant  Value=Flux  OutDataTypeStr=single
  Constant3 : Constant  Value=Ld  OutDataTypeStr=single
  Constant4 : Constant  Value=Lq  OutDataTypeStr=single
  Product{,1..4} (5 alike) : Product
  Subtract : Sum
  Subtract1 : Sum  Inputs=+-
  Torque : Outport
  wires:
  Constant1/1 -> Product/1
  Constant/1 -> Product/2
  Constant2/1 -> Product1/1
  Iq/1 -> Product1/2, Product3/1
  Product1/1 -> Subtract/1
  Constant3/1 -> Subtract1/1
  Constant4/1 -> Subtract1/2
  Subtract1/1 -> Product2/1
  Id/1 -> Product2/2
  Product2/1 -> Product3/2
  Product3/1 -> Subtract/2
  Product/1 -> Product4/1
  Subtract/1 -> Product4/2
  Product4/1 -> Torque/1

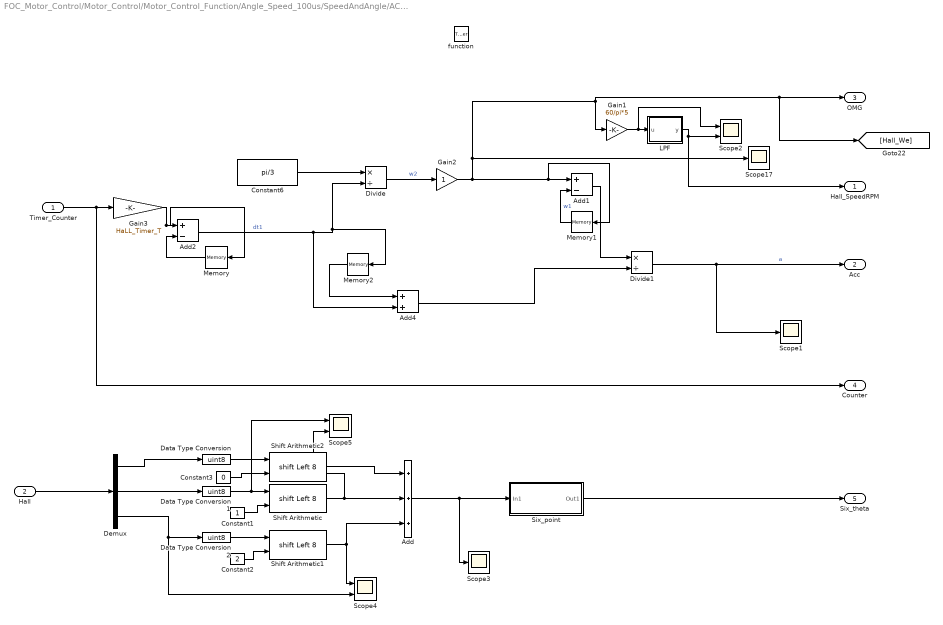
== system FOC_Motor_Control/Motor_Control/Motor_Control_Function/Angle_Speed_100us/SpeedAndAngle/ACC_OMG ==
  Timer_Counter : Inport
  Hall : Inport  Port=2
  function : TriggerPort  TriggerType=either  VariantControl=Variant
  Add : Sum  Inputs=+++
  Add1 : Sum  Inputs=+-
  Add2 : Sum  Inputs=+-
  Add4 : Sum
  Constant1 : Constant  OutDataTypeStr=uint8
  Constant2 : Constant  Value=2  OutDataTypeStr=uint8
  Constant3 : Constant  Value=0  OutDataTypeStr=uint8
  Constant6 : Constant  Value=pi/3  OutDataTypeStr=single
  Data Type Conversion : DataTypeConversion  OutDataTypeStr=uint8
  Data Type Conversion1 : DataTypeConversion  OutDataTypeStr=uint8
  Data Type Conversion2 : DataTypeConversion  OutDataTypeStr=uint8
  Demux : Demux  Outputs=3
  Divide : Product  Inputs=*/
  Divide1 : Product  Inputs=*/
  Gain1 : Gain  Gain=60/pi*5  OutDataTypeStr=Inherit: Same as input  ParamDataTypeStr=Inherit: Same as input
  Gain2 : Gain  OutDataTypeStr=Inherit: Same as input  ParamDataTypeStr=Inherit: Same as input
  Gain3 : Gain  Gain=HaLL_Timer_T
  LPF : Subsystem
  Memory : Memory  InheritSampleTime=on
  Memory1 : Memory  InheritSampleTime=on
  Memory2 : Memory  InheritSampleTime=on
  Scope1 : Scope
  Scope17 : Scope
  Scope2 : Scope  NumInputPorts=2
  Scope3 : Scope
  Scope4 : Scope  NumInputPorts=2
  Scope5 : Scope  NumInputPorts=2
  Shift Arithmetic : ArithShift  BitShiftNumberSource=Input port  BitShiftNumber=8  BitShiftDirection=Left
      settings: InputPortMap=u0,p1
  Shift Arithmetic1 : ArithShift  BitShiftNumberSource=Input port  BitShiftNumber=8  BitShiftDirection=Left
      settings: InputPortMap=u0,p1
  Shift Arithmetic2 : ArithShift  BitShiftNumberSource=Input port  BitShiftNumber=8  BitShiftDirection=Left
      settings: InputPortMap=u0,p1
  Six_point : Subsystem  TreatAsAtomicUnit=on
  Hall_SpeedRPM : Outport
  Acc : Outport  Port=2
  OMG : Outport  Port=3
  Counter : Outport  Port=4
  Six_theta : Outport  Port=5
  wires:
  Timer_Counter/1 -> Counter/1, Gain3/1
  Constant6/1 -> Divide/1
  Divide/1 -> Gain2/1  "w2"
  Memory/1 -> Add2/2
  Add2/1 -> Add4/2, Memory2/1, Divide/2  "dt1"
  Memory1/1 -> Add1/2  "w1"
  Add1/1 -> Divide1/1
  Add4/1 -> Divide1/2
  Divide1/1 -> Acc/1, Scope1/1  "a"
  Gain3/1 -> Memory/1, Add2/1
  Memory2/1 -> Add4/1
  Demux/3 -> Scope4/2, Data Type Conversion2/1
  Data Type Conversion2/1 -> Shift Arithmetic1/1
  Constant2/1 -> Shift Arithmetic1/2
  Constant1/1 -> Shift Arithmetic/2
  Data Type Conversion1/1 -> Scope5/1, Shift Arithmetic/1
  Demux/1 -> Data Type Conversion/1
  Shift Arithmetic/1 -> Add/2, Scope5/2
  Demux/2 -> Data Type Conversion1/1
  Six_point/1(Out1) -> Six_theta/1
  Gain2/1 -> Gain1/1, [Hall_We], OMG/1, Scope17/1, Memory1/1, Add1/1
  Shift Arithmetic1/1 -> Add/3, Scope4/1
  Add/1 -> Scope3/1, Six_point/1(In1)
  Data Type Conversion/1 -> Shift Arithmetic2/1
  Shift Arithmetic2/1 -> Add/1
  Constant3/1 -> Shift Arithmetic2/2
  Hall/1 -> Demux/1
  LPF/1(y) -> Scope2/2, Hall_SpeedRPM/1
  Gain1/1 -> Scope2/1, LPF/1(u)

== system FOC_Motor_Control/Motor_Control/Motor_Control_Function/Angle_Speed_100us/SpeedAndAngle/ADC_IRQ ==
  Counter_ADC_IRQ : Inport
  Acc : Inport  Port=2
  OMG : Inport  Port=3
  Counter_Hall_IRQ : Inport  Port=4
  Six_theta : Inport  Port=5
  Add6 : Sum  Inputs=+-
  Add7 : Sum
  Gain2 : Gain  Gain=HaLL_Timer_T
  Gain3 : Gain  Gain=HaLL_Timer_T
  Gain4 : Gain  Gain=0.5
  Gain5 : Gain
  HallAngle_calibration : Subsystem
      settings: RTWSystemCode=Nonreusable function  RTWFcnNameOpts=Use subsystem name
  Math Function1 : Math  Operator=magnitude^2  SaturateOnIntegerOverflow=on
  Minus2 : Sum
  Product1 : Product
  Product2 : Product
  Hall_Angle : Outport
  wires:
  Gain5/1 -> Minus2/2
  Gain3/1 -> Math Function1/1
  Product2/1 -> Gain4/1
  Counter_Hall_IRQ/1 -> Add6/2
  Gain4/1 -> Minus2/1
  Add6/1 -> Gain3/1, Product1/2
  Math Function1/1 -> Product2/2
  Product1/1 -> Gain2/1
  Gain2/1 -> Gain5/1
  Counter_ADC_IRQ/1 -> Add6/1
  OMG/1 -> Product1/1
  Add7/1 -> HallAngle_calibration/1(Angle_input)
  Minus2/1 -> Add7/1
  Six_theta/1 -> Add7/2
  HallAngle_calibration/1(Angle_output) -> Hall_Angle/1  "SMO_Angle"
  Acc/1 -> Product2/1

== system FOC_Motor_Control/Motor_Control/Motor_Control_Function/Angle_Speed_100us/Speed_Resolver/Speed_cacl ==
  note: Speed_Measured
  position : Inport  OutMin=-4*pi  OutMax=4*pi
      settings: AttributesFormatString="------------------\\nMin =  %<OutMin>\\nMax =  %<OutMax>"
  Constant : Constant  Value=pi/(2^31 -1)/(1/PWM_Frequency)  OutDataTypeStr=single
  Constant1 : Constant  Value=1/Pole_Pairs  OutDataTypeStr=single
  Difference_Wrap : Sum  Inputs=+-  AccumDataTypeStr=int32  OutDataTypeStr=int32
  Difference_to_Single : DataTypeConversion  OutDataTypeStr=single
  Difference_to_Single1 : DataTypeConversion  OutDataTypeStr=int32
  Gain : Gain  Gain=60/(2*pi)
  LPF : Subsystem
  Position_Delay : Delay  DelayLength=1
  Product : Product
  Product1 : Product
  Scale_Input : Gain  Gain=((2^31) - 1)/(4*pi)  ParamDataTypeStr=single  OutDataTypeStr=single
      settings: AttributesFormatString=---------------------------------\n%<Gain>
  Scope : Scope  NumInputPorts=2
  Wrap_To_Pi : Gain  Gain=4  RndMeth=Simplest  OutDataTypeStr=Inherit: Same as input  ParamDataTypeStr=Inherit: Same as input
  Speed_RPM : Outport  VectorParamsAs1DForOutWhenUnconnected=off
  wires:
  position/1 -> Scale_Input/1  "position"
  Difference_to_Single/1 -> Product/2
  Wrap_To_Pi/1 -> Difference_Wrap/1, Position_Delay/1
  Position_Delay/1 -> Difference_Wrap/2
  Scale_Input/1 -> Difference_to_Single1/1
  Difference_Wrap/1 -> Difference_to_Single/1
  Constant/1 -> Product/1
  Constant1/1 -> Product1/1
  Product/1 -> Gain/1  "We"
  Gain/1 -> Product1/2
  Difference_to_Single1/1 -> Wrap_To_Pi/1
  Product1/1 -> Scope/1, LPF/1(u)
  LPF/1(y) -> Scope/2, Speed_RPM/1

== system FOC_Motor_Control/Motor_Control/Motor_Control_Function/Control_Command_2ms/Control_Command_2ms/Speed_PI ==
  Speed_Command : Inport
  Speed_Measured : Inport  Port=2
  Reset : Inport  Port=3
  Action Port : ActionPort  ActionPortLabel=case [ 0 ]:
  SpeedLoop : Subsystem  Commented=on
  Speed_PI : Subsystem
  Iq_ref : Outport  VectorParamsAs1DForOutWhenUnconnected=off
  wires:
  Speed_PI/1(PI_out) -> Iq_ref/1
  Speed_Command/1 -> Speed_PI/1(Ref)
  Reset/1 -> Speed_PI/3(Reset)
  Speed_Measured/1 -> Speed_PI/2(Fdk)

== system FOC_Motor_Control/Motor_Control/Motor_Control_Function/Control_Command_2ms/Control_Command_2ms/Switch Case Action Subsystem ==
  Iq_in : Inport
  Action Port : ActionPort  ActionPortLabel=case [ 1 ]:
  Iq_out : Outport
  wires:
  Iq_in/1 -> Iq_out/1

== system FOC_Motor_Control/Motor_Control/Motor_Control_Function/Control_Command_2ms/Subsystem/Hall_Spd ==
  Hall_Speed : Inport
  Action Port : ActionPort  ActionPortLabel=elseif(u1==0)
  Out1 : Outport
  wires:
  Hall_Speed/1 -> Out1/1

== system FOC_Motor_Control/Motor_Control/Motor_Control_Function/Control_Command_2ms/Subsystem/Obs_Spd ==
  Obs_Speed : Inport
  Action Port : ActionPort  ActionPortLabel=if(u1==1)
  Out1 : Outport
  wires:
  Obs_Speed/1 -> Out1/1

== system FOC_Motor_Control/Motor_Control/Motor_Control_Function/FOC_Control_100us/FOC/Clarke_Transform ==
  Phase_CurrentABC : Inport  PortDimensions=3
  Clark1 : Subsystem  TreatAsAtomicUnit=on
  Scope : Scope  NumInputPorts=2
  IAlpha : Outport  VectorParamsAs1DForOutWhenUnconnected=off
  IBeta : Outport  Port=2  VectorParamsAs1DForOutWhenUnconnected=off
  wires:
  Clark1/1(Ialpha) -> IAlpha/1, Scope/1
  Clark1/2(Ibeta) -> IBeta/1, Scope/2
  Phase_CurrentABC/1 -> Clark1/1(Iabc)

== system FOC_Motor_Control/Motor_Control/Motor_Control_Function/FOC_Control_100us/FOC/D_Current_PI ==
  Reset : Inport
  Bus_voltage : Inport  Port=2
  Current_Command : Inport  Port=3
  Current_Measured : Inport  Port=4
  Add2 : Sum  Inputs=|+-
  ID_Control : Subsystem
  Vd_voltage : Outport  VectorParamsAs1DForOutWhenUnconnected=off
  wires:
  Current_Command/1 -> Add2/1
  Current_Measured/1 -> Add2/2
  Add2/1 -> ID_Control/3(Err)  "currentControlError"
  Reset/1 -> ID_Control/1(Reset)
  Bus_voltage/1 -> ID_Control/2(Bus_voltage)
  ID_Control/1(PI_Out) -> Vd_voltage/1

== system FOC_Motor_Control/Motor_Control/Motor_Control_Function/FOC_Control_100us/FOC/Flux_Observer ==
  Enable : Inport
  i_alpha : Inport  Port=2  OutDataTypeStr=single
  i_beta : Inport  Port=3  OutDataTypeStr=single
  u_alpha : Inport  Port=4  OutDataTypeStr=single
  u_beta : Inport  Port=5  OutDataTypeStr=single
  Gain{,1..3} (4 alike) : Gain  Gain=Flux_Gain
  OBSERVER : Subsystem
  Scope : Scope  NumInputPorts=2
  Scope1 : Scope  NumInputPorts=2
  Obs_Theta : Outport
  Obs_Speed : Outport  Port=2
  wires:
  i_beta/1 -> Scope1/2, Gain1/1
  u_alpha/1 -> Scope/1, Gain2/1
  u_beta/1 -> Scope/2, Gain3/1
  i_alpha/1 -> Scope1/1, Gain/1
  Gain/1 -> OBSERVER/1(i_alpha)
  Gain1/1 -> OBSERVER/2(i_beta)
  Gain2/1 -> OBSERVER/3(u_alpha)
  Gain3/1 -> OBSERVER/4(u_beta)
  OBSERVER/1(Obs_Theta) -> Obs_Theta/1
  OBSERVER/2(Obs_Speed) -> Obs_Speed/1

== system FOC_Motor_Control/Motor_Control/Motor_Control_Function/FOC_Control_100us/FOC/Hall_Angle ==
  Hall_Angle : Inport
  Action Port : ActionPort  ActionPortLabel=elseif(u1==0)
  Out1 : Outport
  wires:
  Hall_Angle/1 -> Out1/1
